simulink model "Resistor_Models"  (R2021b)
settings: Solver=VariableStepAuto  StartTime=0.0  StopTime=10.0  RelTol=1e-3
libraries: nesl_utility x14, fl_lib x12, ee_lib x4, spspowerguiLib x1
settings Model: Creator=josec  LastModifiedBy=josec

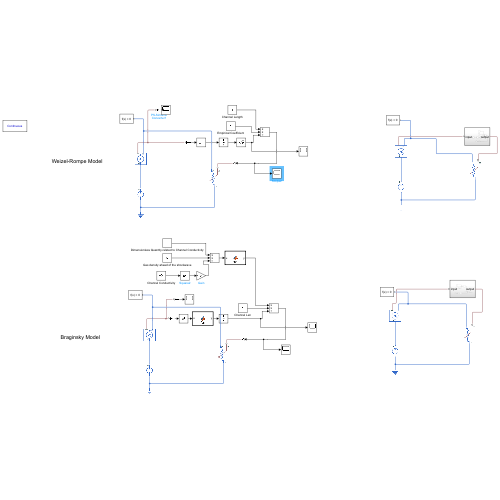
[thumbnail: Simulink's stored preview of the top-level diagram]
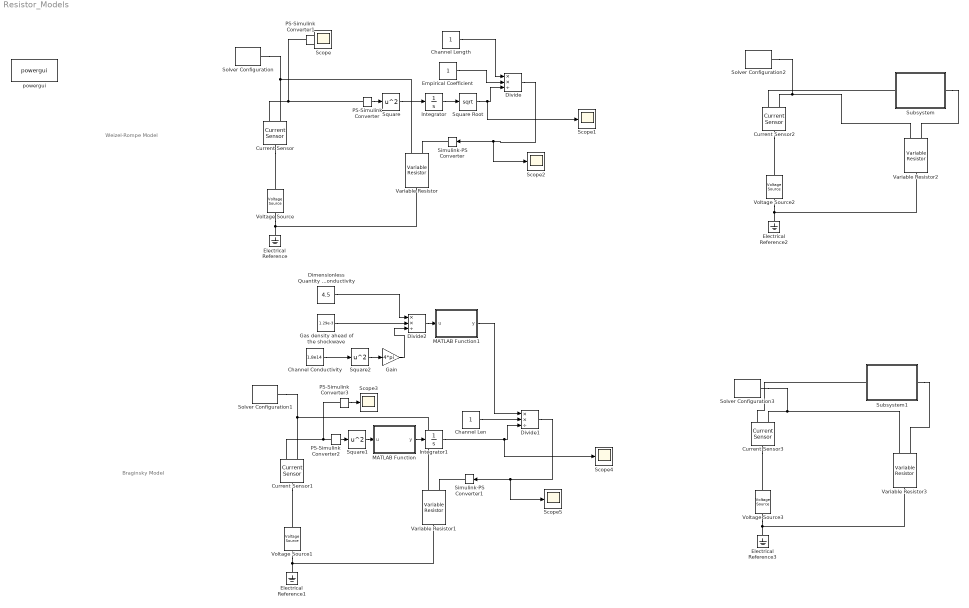
== system Resistor_Models ==
  note: Weizel-Rompe Model
  note: Braginsky Model
  Channel Conductivity : Constant  Value=1.8e14
  Channel Len : Constant
  Channel Length : Constant
  Current Sensor{,1..3} (4 alike) : fl_lib/Electrical/Electrical Sensors/Current Sensor
  Dimensionless Quantity related to Channel Conductivity : Constant  Value=4.5
  Divide : Product  Inputs=**/
  Divide1 : Product  Inputs=**/
  Divide2 : Product  Inputs=**/
  Electrical Reference{,1..3} (4 alike) : fl_lib/Electrical/Electrical Elements/Electrical Reference
  Empirical Coefficient : Constant
  Gain : Gain  Gain=4*pi
  Gas density ahead of the shockwave : Constant  Value=1.29e-3
  Integrator : Integrator  InitialCondition=1e-36
  Integrator1 : Integrator  InitialCondition=1e-36
  MATLAB Function : MATLAB Function  TreatAsAtomicUnit=on
  MATLAB Function1 : MATLAB Function  TreatAsAtomicUnit=on
  PS-Simulink Converter{,1..3} (4 alike) : nesl_utility/PS-Simulink Converter  PhysicalDomain=network_engine_domain  SubClassName=ps_output  LeftPortType=input  RightPortType=output  PseudoPeriodic=off  Frequencies=[]  Unit=inherit  AffineConversion=off
      settings: SourceProductBaseCode=PW,SS
  Scope{,1..5} (6 alike) : Scope
  Simulink-PS Converter : nesl_utility/Simulink-PS Converter  PhysicalDomain=network_engine_domain  SubClassName=ps_input  LeftPortType=input  RightPortType=output  PseudoPeriodic=off  Frequencies=[]  NoiseDistribution=none  NoiseParameters=[]  Unit=1  AffineConversion=off  FilteringAndDerivatives=provide  SimscapeFilterOrder=1  InputFilterTimeConstant=0.001  UdotUserProvided=0
      settings: SourceProductBaseCode=PW,SS
  Simulink-PS Converter1 : nesl_utility/Simulink-PS Converter  PhysicalDomain=network_engine_domain  SubClassName=ps_input  LeftPortType=input  RightPortType=output  PseudoPeriodic=off  Frequencies=[]  NoiseDistribution=none  NoiseParameters=[]  Unit=1  AffineConversion=off  FilteringAndDerivatives=provide  SimscapeFilterOrder=1  InputFilterTimeConstant=0.001  UdotUserProvided=0
      settings: SourceProductBaseCode=PW,SS
  Solver Configuration{,1..3} (4 alike) : nesl_utility/Solver Configuration  PhysicalDomain=network_engine_domain  SubClassName=solver  LeftPortType=input  RightPortType=generic  Tones=[]  Harmonics=[]  SimulateNoise=off  Profile=off  UseLocalSampling=off  EnableSwitchedLinearOptims=on  FrequencyDomain=off  UseCCode=off  RelTol=0.001  AbsTol=1e-06  MinStep=1e-09  ToWorkspace=off  RevertToSquareIcSolve=off  NumHomotopyIterations=100  PhasorMode=off  PhasorModeNumHarmonics=1  DoDC=off  ResidualTolerance=1e-09  UseLocalSolver=off  LocalSolverChoice=NE_BACKWARD_EULER_ADVANCER  LocalSolverSampleTime=0.001  DoFixedCost=off  MaxNonlinIter=3  MaxModeIter=2  ComputeImpulses=off  ImpulseIterations=2  LinearAlgebra=auto  EquationFormulation=NE_TIME_EF  DelaysMemoryBudget=1024  AutomaticFiltering=on  FilteringTimeConstant=0.001  PartitionStorageMethod=AS_NEEDED  PartitionMemoryBudget=1024  PartitionMethod=ROBUST
      settings: SourceProductBaseCode=PW,SS
  Square : Math  Operator=square  SaturateOnIntegerOverflow=on
  Square Root : Sqrt  SaturateOnIntegerOverflow=on
  Square1 : Math  Operator=square  SaturateOnIntegerOverflow=on
  Square2 : Math  Operator=square  SaturateOnIntegerOverflow=on
  Subsystem : Subsystem
  Subsystem1 : Subsystem
  Variable Resistor{,1..3} (4 alike) : fl_lib/Electrical/Electrical Elements/Variable Resistor  Rmin=1 Ohm  i_specify=off  i_priority=None  i=0 A  i_nominal_specify=off  i_nominal_unit=A  i_nominal_value=1  v_specify=off  v_priority=None  v=0 V  v_nominal_specify=off  v_nominal_unit=V  v_nominal_value=1
  Voltage Source : ee_lib/Sources/Voltage Source  dc_voltage=20 V  ac_voltage=0 V  ac_shift=0 rad  ac_frequency=0 Hz  noise_mode=0  PSD=0 V^2/Hz  repeatability=1  auto_seed=1884392676  user_seed=0  sample_time=1e-3 s  i_specify=off  i_priority=None  i=0 A  i_nominal_specify=off  i_nominal_unit=A  i_nominal_value=1  v_specify=off  v_priority=None  v=0 V  v_nominal_specify=off  v_nominal_unit=V  v_nominal_value=1
  Voltage Source1 : ee_lib/Sources/Voltage Source  dc_voltage=20 V  ac_voltage=0 V  ac_shift=0 rad  ac_frequency=0 Hz  noise_mode=0  PSD=0 V^2/Hz  repeatability=1  auto_seed=1315760964  user_seed=0  sample_time=1e-3 s  i_specify=off  i_priority=None  i=0 A  i_nominal_specify=off  i_nominal_unit=A  i_nominal_value=1  v_specify=off  v_priority=None  v=0 V  v_nominal_specify=off  v_nominal_unit=V  v_nominal_value=1
  Voltage Source2 : ee_lib/Sources/Voltage Source  dc_voltage=20 V  ac_voltage=0 V  ac_shift=0 rad  ac_frequency=0 Hz  noise_mode=0  PSD=0 V^2/Hz  repeatability=1  auto_seed=3626278652  user_seed=0  sample_time=1e-3 s  i_specify=off  i_priority=None  i=0 A  i_nominal_specify=off  i_nominal_unit=A  i_nominal_value=1  v_specify=off  v_priority=None  v=0 V  v_nominal_specify=off  v_nominal_unit=V  v_nominal_value=1
  Voltage Source3 : ee_lib/Sources/Voltage Source  dc_voltage=20 V  ac_voltage=0 V  ac_shift=0 rad  ac_frequency=0 Hz  noise_mode=0  PSD=0 V^2/Hz  repeatability=1  auto_seed=836506254  user_seed=0  sample_time=1e-3 s  i_specify=off  i_priority=None  i=0 A  i_nominal_specify=off  i_nominal_unit=A  i_nominal_value=1  v_specify=off  v_priority=None  v=0 V  v_nominal_specify=off  v_nominal_unit=V  v_nominal_value=1
  powergui : spspowerguiLib/powergui  Priority=1  SimulationMode=Continuous  SampleTime=50e-6  frequency=60  Iterations=50  frequencyindice=60  Pbase=100e6  ErrMax=1e-4  UnitsV=kV  UnitsW=MW  buscounter=0  FunctionMessages=off  echomessages=off  EnableUseOfTLC=off  CurrentSourceSwitches=off  DisableSnubberDevices=off  DisableRonSwitches=off  DisableVfSwitches=off  DisplayEquations=off  AutomaticDiscreteSolvers=off  SolverType=Tustin/Backward Euler (TBE)  Interpol=off  ExternalGateDelay=off  methode=off  Ts=100  x0status=blocks  SPID=on  SwTol=0  HookPort=off  NonlinearTolerance=1e-4  nMaxIteration=100  ContinueOnMaxIteration=off  RestoreLinks=warning  ResistiveCurrentMeasurement=off  Frange=[0:2:500]  Ylog=off  Xlog=on  ShowGrid=off  save=off  variable=ZData  structure=0  ZoomFFT=off  StartTime=0.0  cycles=1  DisplayStyle=1  fundamental=60  FreqAxis=off  MaxFrequency=1000  frequencyindicesteady=1  RmsSteady=1  display=off
  wires:
  Square/1 -> Integrator/1
  PS-Simulink Converter/1 -> Square/1
  Integrator/1 -> Square Root/1
  Empirical Coefficient/1 -> Divide/2
  Channel Length/1 -> Divide/1
  PS-Simulink Converter1/1 -> Scope/1
  Square Root/1 -> Scope1/1, Divide/3
  Divide/1 -> Scope2/1, Simulink-PS Converter/1
  Square1/1 -> MATLAB Function/1(u)
  Divide1/1 -> Scope5/1, Simulink-PS Converter1/1
  PS-Simulink Converter3/1 -> Scope3/1
  Channel Len/1 -> Divide1/2
  PS-Simulink Converter2/1 -> Square1/1
  Integrator1/1 -> Scope4/1, Divide1/3
  MATLAB Function1/1(y) -> Divide1/1
  MATLAB Function/1(y) -> Integrator1/1
  Divide2/1 -> MATLAB Function1/1(u)
  Dimensionless Quantity related to Channel Conductivity/1 -> Divide2/1
  Gas density ahead of the shockwave/1 -> Divide2/2
  Channel Conductivity/1 -> Square2/1
  Square2/1 -> Gain/1
  Gain/1 -> Divide2/3
  connections:
  Current Sensor/LConn1 -- Voltage Source/LConn1
  PS-Simulink Converter/LConn1 -- PS-Simulink Converter1/LConn1 -- Current Sensor/RConn1
  Variable Resistor/LConn1 -- Simulink-PS Converter/RConn1
  Variable Resistor/LConn2 -- Current Sensor/RConn2 -- Solver Configuration/RConn1
  Voltage Source/RConn1 -- Electrical Reference/LConn1 -- Variable Resistor/RConn1
  Variable Resistor1/RConn1 -- Voltage Source1/RConn1 -- Electrical Reference1/LConn1
  PS-Simulink Converter2/LConn1 -- PS-Simulink Converter3/LConn1 -- Current Sensor1/RConn1
  Variable Resistor1/LConn2 -- Current Sensor1/RConn2 -- Solver Configuration1/RConn1
  Current Sensor1/LConn1 -- Voltage Source1/LConn1
  Variable Resistor1/LConn1 -- Simulink-PS Converter1/RConn1
  Variable Resistor2/RConn1 -- Voltage Source2/RConn1 -- Electrical Reference2/LConn1
  Current Sensor2/LConn1 -- Voltage Source2/LConn1
  Current Sensor2/RConn2 -- Solver Configuration2/RConn1 -- Variable Resistor2/LConn2
  Subsystem/LConn1 -- Current Sensor2/RConn1
  Subsystem/RConn1 -- Variable Resistor2/LConn1
  Variable Resistor3/RConn1 -- Voltage Source3/RConn1 -- Electrical Reference3/LConn1
  Current Sensor3/LConn1 -- Voltage Source3/LConn1
  Current Sensor3/RConn2 -- Solver Configuration3/RConn1 -- Variable Resistor3/LConn2
  Current Sensor3/RConn1 -- Subsystem1/LConn1
  Subsystem1/RConn1 -- Variable Resistor3/LConn1

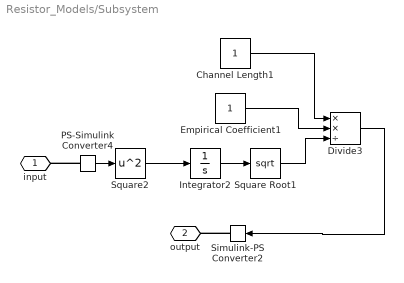
== system Resistor_Models/Subsystem ==
  Channel Length1 : Constant
  Divide3 : Product  Inputs=**/
  Empirical Coefficient1 : Constant
  Integrator2 : Integrator  InitialCondition=1e-36
  PS-Simulink Converter4 : nesl_utility/PS-Simulink Converter  PhysicalDomain=network_engine_domain  SubClassName=ps_output  LeftPortType=input  RightPortType=output  PseudoPeriodic=off  Frequencies=[]  Unit=inherit  AffineConversion=off
      settings: SourceProductBaseCode=PW,SS
  Simulink-PS Converter2 : nesl_utility/Simulink-PS Converter  PhysicalDomain=network_engine_domain  SubClassName=ps_input  LeftPortType=input  RightPortType=output  PseudoPeriodic=off  Frequencies=[]  NoiseDistribution=none  NoiseParameters=[]  Unit=1  AffineConversion=off  FilteringAndDerivatives=provide  SimscapeFilterOrder=1  InputFilterTimeConstant=0.001  UdotUserProvided=0
      settings: SourceProductBaseCode=PW,SS
  Square Root1 : Sqrt  SaturateOnIntegerOverflow=on
  Square2 : Math  Operator=square  SaturateOnIntegerOverflow=on
  input : PMIOPort  Side=Left
  output : PMIOPort  Port=2  Side=Right
  wires:
  Square Root1/1 -> Divide3/3
  Integrator2/1 -> Square Root1/1
  Empirical Coefficient1/1 -> Divide3/2
  PS-Simulink Converter4/1 -> Square2/1
  Channel Length1/1 -> Divide3/1
  Divide3/1 -> Simulink-PS Converter2/1
  Square2/1 -> Integrator2/1
  connections:
  Simulink-PS Converter2/RConn1 -- output/RConn1
  PS-Simulink Converter4/LConn1 -- input/RConn1

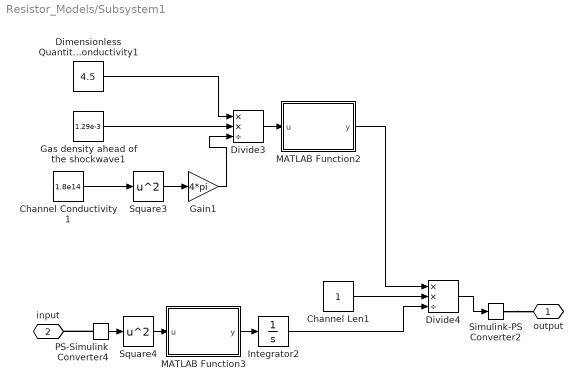
== system Resistor_Models/Subsystem1 ==
  Channel Conductivity1 : Constant  Value=1.8e14
  Channel Len1 : Constant
  Dimensionless Quantity related to Channel Conductivity1 : Constant  Value=4.5
  Divide3 : Product  Inputs=**/
  Divide4 : Product  Inputs=**/
  Gain1 : Gain  Gain=4*pi
  Gas density ahead of the shockwave1 : Constant  Value=1.29e-3
  Integrator2 : Integrator  InitialCondition=1e-36
  MATLAB Function2 : MATLAB Function  TreatAsAtomicUnit=on
  MATLAB Function3 : MATLAB Function  TreatAsAtomicUnit=on
  PS-Simulink Converter4 : nesl_utility/PS-Simulink Converter  PhysicalDomain=network_engine_domain  SubClassName=ps_output  LeftPortType=input  RightPortType=output  PseudoPeriodic=off  Frequencies=[]  Unit=inherit  AffineConversion=off
      settings: SourceProductBaseCode=PW,SS
  Simulink-PS Converter2 : nesl_utility/Simulink-PS Converter  PhysicalDomain=network_engine_domain  SubClassName=ps_input  LeftPortType=input  RightPortType=output  PseudoPeriodic=off  Frequencies=[]  NoiseDistribution=none  NoiseParameters=[]  Unit=1  AffineConversion=off  FilteringAndDerivatives=provide  SimscapeFilterOrder=1  InputFilterTimeConstant=0.001  UdotUserProvided=0
      settings: SourceProductBaseCode=PW,SS
  Square3 : Math  Operator=square  SaturateOnIntegerOverflow=on
  Square4 : Math  Operator=square  SaturateOnIntegerOverflow=on
  output : PMIOPort  Side=Right
  input : PMIOPort  Port=2  Side=Left
  wires:
  PS-Simulink Converter4/1 -> Square4/1
  Dimensionless Quantity related to Channel Conductivity1/1 -> Divide3/1
  MATLAB Function2/1(y) -> Divide4/1
  Channel Len1/1 -> Divide4/2
  Divide3/1 -> MATLAB Function2/1(u)
  Gain1/1 -> Divide3/3
  Gas density ahead of the shockwave1/1 -> Divide3/2
  Square3/1 -> Gain1/1
  Channel Conductivity1/1 -> Square3/1
  Integrator2/1 -> Divide4/3
  Square4/1 -> MATLAB Function3/1(u)
  MATLAB Function3/1(y) -> Integrator2/1
  Divide4/1 -> Simulink-PS Converter2/1
  connections:
  PS-Simulink Converter4/LConn1 -- input/RConn1
  Simulink-PS Converter2/RConn1 -- output/RConn1

== matlab function Resistor_Models/MATLAB Function ==
  data: u input; y output
function y = fcn(u)

y = u^(1/3);

== matlab function Resistor_Models/Subsystem1/MATLAB Function2 ==
  data: u input; y output
function y = fcn(u)

y = u^(1/3);

== matlab function Resistor_Models/Subsystem1/MATLAB Function3 ==
  data: u input; y output
function y = fcn(u)

y = u^(1/3);

== matlab function Resistor_Models/MATLAB Function1 ==
  data: u input; y output
function y = fcn(u)

y = u^(1/3);
